simulink model "model"  (R2018a)
settings: Solver=VariableStepAuto  StartTime=0.0  StopTime=20  MaxStep=0.01  RelTol=1e-8  EnableMultiTasking=on
settings Model: Creator=Pracownik  LastModifiedBy=CHADI
settings DataIOCC: LimitDataPoints=on
settings OptimizationCC: LifeSpan=inf
settings DebuggingCC: AllowSymbolicDim=off  SFUnexpectedBacktrackingDiag=warning  SFNoUnconditionalDefaultTransitionDiag=warning  SFExecutionAtInitializationDiag=none
settings ModelReferenceCC: PropagateSignalLabelsOutOfModel=off
settings CodeAppCC: StateflowObjectComments=on
settings GRTTargetCC: TargetLangStandard=C89/C90 (ANSI)
settings ConfigComp: CovMetricSettings=dw  CovHtmlReporting=on  CovSaveCumulativeToWorkspaceVar=on  CovSaveSingleToWorkspaceVar=on  CovExternalEMLEnable=off

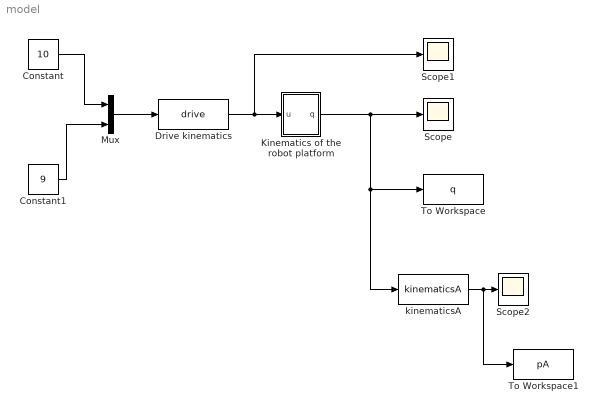
== system model ==
  Constant : Constant  Value=10
  Constant1 : Constant  Value=9
  Drive kinematics : MATLABFcn  MATLABFcn=drive
  Kinematics of the robot platform : Subsystem
  Mux : Mux  Inputs=2
  Scope : Scope
  Scope1 : Scope
  Scope2 : Scope
  To Workspace : ToWorkspace  VariableName=q  SampleTime=-1
  To Workspace1 : ToWorkspace  VariableName=pA  SampleTime=-1
  kinematicsA : MATLABFcn  MATLABFcn=kinematicsA
  wires:
  Kinematics of the robot platform/1(q) -> Scope/1, kinematicsA/1, To Workspace/1
  Mux/1 -> Drive kinematics/1
  Constant/1 -> Mux/1
  Constant1/1 -> Mux/2
  Drive kinematics/1 -> Scope1/1, Kinematics of the robot platform/1(u)
  kinematicsA/1 -> To Workspace1/1, Scope2/1

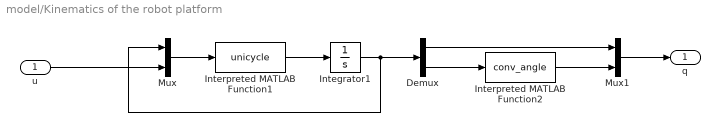
== system model/Kinematics of the robot platform ==
  u : Inport
  Demux : Demux  Outputs=[2 1]
  Integrator1 : Integrator  InitialCondition=[0; 0; 0]
  Interpreted MATLAB Function1 : MATLABFcn  MATLABFcn=unicycle
  Interpreted MATLAB Function2 : MATLABFcn  MATLABFcn=conv_angle
  Mux : Mux  Inputs=[3 2]
  Mux1 : Mux  Inputs=[2 1]
  q : Outport
  wires:
  Mux/1 -> Interpreted MATLAB Function1/1
  Interpreted MATLAB Function1/1 -> Integrator1/1
  Integrator1/1 -> Demux/1, Mux/1
  u/1 -> Mux/2
  Demux/2 -> Interpreted MATLAB Function2/1
  Interpreted MATLAB Function2/1 -> Mux1/2
  Demux/1 -> Mux1/1
  Mux1/1 -> q/1
